simulink model "G2"  (R2023b)
settings: Solver=VariableStepAuto  StartTime=0.0  StopTime=0.2  RelTol=1e-3
undefined symbols (not defined in the file or in its folder): b, f_final, f_inicial, fa, k, m, t_inicial
settings Model: Creator=klaus  LastModifiedBy=thiag
settings SolverCC: AlgebraicLoopSolver=TrustRegion
settings DebuggingCC: UnconnectedInputMsg=warning  UnconnectedOutputMsg=warning  UnconnectedLineMsg=warning
settings ModelReferenceCC: EnableRefExpFcnMdlSchedulingChecks=on

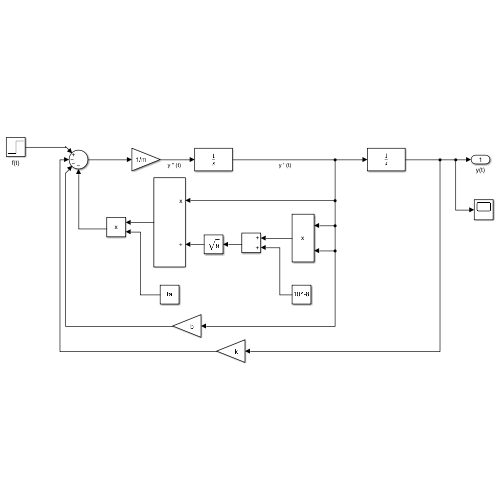
[thumbnail: Simulink's stored preview of the top-level diagram]
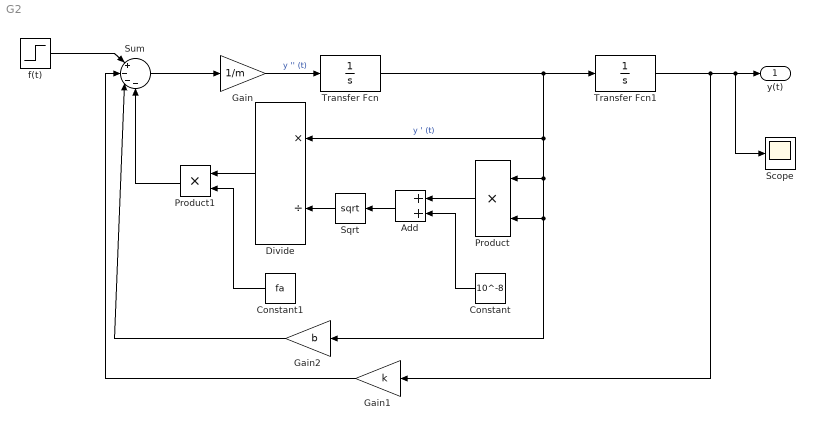
== system G2 ==
  Add : Sum
  Constant : Constant  Value=10^-8
  Constant1 : Constant  Value=fa
  Divide : Product  Inputs=*/
  Gain : Gain  Gain=1/m
  Gain1 : Gain  Gain=k
  Gain2 : Gain  Gain=b
  Product : Product
  Product1 : Product
  Scope : Scope
  Sqrt : Sqrt
  Sum : Sum  Inputs=|+---
  Transfer Fcn : TransferFcn  Denominator=[1 0]
  Transfer Fcn1 : TransferFcn  Denominator=[1 0]
  f(t) : Step  Time=t_inicial  Before=f_inicial  After=f_final  SampleTime=0
  y(t) : Outport
  wires:
  Gain/1 -> Transfer Fcn/1  "y '' (t)"
  f(t)/1 -> Sum/1
  Transfer Fcn/1 -> Gain2/1, Product/2, Product/1, Divide/1, Transfer Fcn1/1  "y ' (t)"
  Gain2/1 -> Sum/3
  Sum/1 -> Gain/1
  Transfer Fcn1/1 -> Gain1/1, Scope/1, y(t)/1
  Gain1/1 -> Sum/2
  Divide/1 -> Product1/1
  Sqrt/1 -> Divide/2
  Product/1 -> Add/1
  Add/1 -> Sqrt/1
  Constant/1 -> Add/2
  Constant1/1 -> Product1/2
  Product1/1 -> Sum/4
